simulink library "Phase2_Kinematics_Lib"  (R2026a)
settings: Solver=VariableStepAuto
settings Model: Creator=shueb  LastModifiedBy=shueb

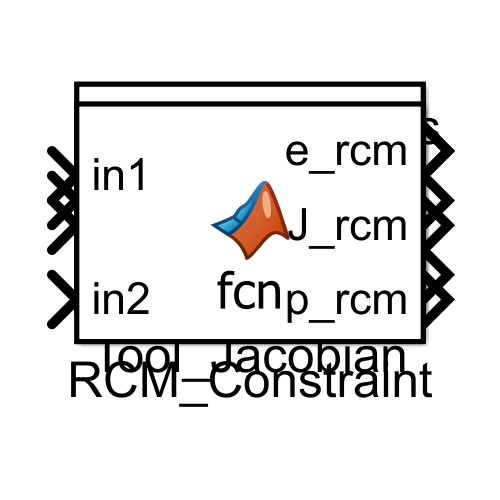
[thumbnail: Simulink's stored preview of the top-level diagram]
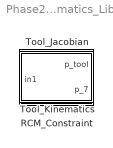
== system Phase2_Kinematics_Lib ==
  RCM_Constraint : MATLAB Function  TreatAsAtomicUnit=on
  Tool_Jacobian : MATLAB Function  TreatAsAtomicUnit=on
  Tool_Kinematics : MATLAB Function  TreatAsAtomicUnit=on

== matlab function Phase2_Kinematics_Lib/Tool_Jacobian ==
  data: in1 input; J_tool output
function J_tool = tool_jacobian(in1)
%#codegen

%    This function was generated by the Symbolic Math Toolbox version 26.1.
%    26-May-2026 08:31:23

% in1 = complex(in1);  % if required to enforce complex operations
q1 = in1(1,:);
q2 = in1(2,:);
q3 = in1(3,:);
q4 = in1(4,:);
q5 = in1(5,:);
q6 = in1(6,:);
t2 = cos(q1);
t3 = cos(q2);
t4 = cos(q3);
t5 = cos(q4);
t6 = cos(q5);
t7 = cos(q6);
t8 = sin(q1);
t9 = sin(q2);
t10 = sin(q3);
t11 = sin(q4);
t12 = sin(q5);
t13 = sin(q6);
t14 = t2.*t4;
t15 = t3.*t5;
t16 = t2.*t10;
t17 = t4.*t8;
t18 = t3.*t11;
t19 = t8.*t10;
t20 = t8.*t9.*t11;
t24 = t2.*t5.*t9;
t25 = t4.*t5.*t9;
t27 = t2.*t9.*t11;
t28 = t5.*t8.*t9;
t29 = t4.*t9.*t11;
t21 = t3.*t14;
t22 = t3.*t16;
t23 = t3.*t17;
t26 = t3.*t19;
t31 = -t25;
t37 = t15+t29;
t30 = -t21;
t32 = -t26;
t35 = t16+t23;
t36 = t17+t22;
t40 = t18+t31;
t38 = t14+t32;
t39 = t19+t30;
t41 = t5.*t35;
t42 = t11.*t35;
t43 = t12.*t36;
t44 = t5.*t39;
t45 = t11.*t39;
t46 = t12.*t38;
t47 = t20+t41;
t49 = t24+t45;
t50 = t6.*t47;
t52 = -t6.*(t27-t44);
t53 = t46+t50;
t54 = t43+t52;
mt1 = [t28.*(2.0./5.0)-t42.*(2.0./5.0)+t8.*t9.*(2.0./5.0)+t13.*t53.*(6.9e+1./2.5e+2)+t7.*(t28-t42).*(6.9e+1./2.5e+2),t24.*(-2.0./5.0)-t45.*(2.0./5.0)-t2.*t9.*(2.0./5.0)-t7.*t49.*(6.9e+1./2.5e+2)+t13.*t54.*(6.9e+1./2.5e+2),0.0,t13.*(t6.*(t2.*t18-t5.*t9.*t14)+t9.*t12.*t16).*(-6.9e+1./2.5e+2)-t7.*(t2.*t15+t9.*t11.*t14).*(6.9e+1./2.5e+2)-t2.*t3.*(2.0./5.0)-t2.*t15.*(2.0./5.0)-t9.*t11.*t14.*(2.0./5.0)];
mt2 = [t13.*(t6.*(t8.*t18-t5.*t9.*t17)+t9.*t12.*t19).*(-6.9e+1./2.5e+2)-t7.*(t8.*t15+t9.*t11.*t17).*(6.9e+1./2.5e+2)-t3.*t8.*(2.0./5.0)-t8.*t15.*(2.0./5.0)-t9.*t11.*t17.*(2.0./5.0),t9.*(-2.0./5.0)-t5.*t9.*(2.0./5.0)+t4.*t18.*(2.0./5.0)-t13.*(t6.*(t4.*t15+t9.*t11)-t3.*t10.*t12).*(6.9e+1./2.5e+2)-t7.*(t5.*t9-t4.*t18).*(6.9e+1./2.5e+2),t13.*(t12.*t39-t5.*t6.*t36).*(-6.9e+1./2.5e+2)-t11.*t36.*(2.0./5.0)-t7.*t11.*t36.*(6.9e+1./2.5e+2)];
mt3 = [t13.*(t12.*t35-t5.*t6.*t38).*(6.9e+1./2.5e+2)+t11.*t38.*(2.0./5.0)+t7.*t11.*t38.*(6.9e+1./2.5e+2),t13.*(t4.*t9.*t12+t5.*t6.*t9.*t10).*(6.9e+1./2.5e+2)-t9.*t10.*t11.*(2.0./5.0)-t7.*t9.*t10.*t11.*(6.9e+1./2.5e+2),t27.*(2.0./5.0)-t44.*(2.0./5.0)+t7.*(t27-t44).*(6.9e+1./2.5e+2)-t6.*t13.*t49.*(6.9e+1./2.5e+2),t20.*(2.0./5.0)+t41.*(2.0./5.0)+t7.*t47.*(6.9e+1./2.5e+2)-t6.*t13.*(t28-t42).*(6.9e+1./2.5e+2),t18.*(-2.0./5.0)+t25.*(2.0./5.0)-t7.*t40.*(6.9e+1./2.5e+2)+t6.*t13.*t37.*(6.9e+1./2.5e+2)];
mt4 = [t13.*(t6.*t36+t12.*(t27-t44)).*(6.9e+1./2.5e+2),t13.*(t6.*t38-t12.*t47).*(-6.9e+1./2.5e+2),t13.*(t12.*t40-t6.*t9.*t10).*(-6.9e+1./2.5e+2),t7.*t54.*(6.9e+1./2.5e+2)+t13.*t49.*(6.9e+1./2.5e+2),t7.*t53.*(-6.9e+1./2.5e+2)+t13.*(t28-t42).*(6.9e+1./2.5e+2),t7.*(t6.*t40+t9.*t10.*t12).*(6.9e+1./2.5e+2)-t13.*t37.*(6.9e+1./2.5e+2),0.0,0.0,0.0];
J_tool = reshape([mt1,mt2,mt3,mt4],3,7);
end

== matlab function Phase2_Kinematics_Lib/Tool_Kinematics ==
  data: in1 input; p_tool output; p_7 output
function [p_tool,p_7] = tool_kinematics(in1)
%#codegen

%    This function was generated by the Symbolic Math Toolbox version 26.1.
%    26-May-2026 08:31:21

% in1 = complex(in1);  % if required to enforce complex operations
q1 = in1(1,:);
q2 = in1(2,:);
q3 = in1(3,:);
q4 = in1(4,:);
q5 = in1(5,:);
q6 = in1(6,:);
t2 = cos(q1);
t3 = cos(q2);
t4 = cos(q3);
t5 = cos(q4);
t6 = cos(q5);
t7 = cos(q6);
t8 = sin(q1);
t9 = sin(q2);
t10 = sin(q3);
t11 = sin(q4);
t12 = sin(q5);
t13 = sin(q6);
t14 = t2.*t4;
t15 = t3.*t5;
t16 = t2.*t10;
t17 = t4.*t8;
t18 = t3.*t11;
t19 = t8.*t10;
t20 = t3.*(2.0./5.0);
t21 = t8.*t9.*t11;
t22 = t9.*t10.*t12;
t26 = t2.*t5.*t9;
t27 = t4.*t5.*t9;
t29 = t2.*t9.*t11;
t30 = t5.*t8.*t9;
t31 = t4.*t9.*t11;
t33 = t2.*t9.*(2.0./5.0);
t34 = t8.*t9.*(2.0./5.0);
t23 = t3.*t14;
t24 = t3.*t16;
t25 = t3.*t17;
t28 = t3.*t19;
t32 = t15.*(2.0./5.0);
t35 = -t33;
t36 = -t34;
t38 = -t27;
t42 = t26.*(2.0./5.0);
t43 = t30.*(2.0./5.0);
t44 = t31.*(2.0./5.0);
t49 = t15+t31;
t37 = -t23;
t39 = -t28;
t45 = -t42;
t46 = -t43;
t47 = t16+t25;
t48 = t17+t24;
t52 = t18+t38;
t50 = t14+t39;
t51 = t19+t37;
t53 = t5.*t47;
t54 = t11.*t47;
t55 = t12.*t48;
t57 = t6.*t52;
t56 = t5.*t51;
t58 = t11.*t51;
t59 = t12.*t50;
t60 = t54.*(2.0./5.0);
t63 = t21+t53;
t65 = t22+t57;
t61 = t58.*(2.0./5.0);
t66 = t26+t58;
t67 = t6.*t63;
t69 = -t6.*(t29-t56);
t62 = -t61;
t70 = t59+t67;
t71 = t55+t69;
p_tool = [t35+t45+t62-t7.*t66.*(6.9e+1./2.5e+2)+t13.*t71.*(6.9e+1./2.5e+2);t36+t46+t60-t13.*t70.*(6.9e+1./2.5e+2)-t7.*(t30-t54).*(6.9e+1./2.5e+2);t20+t32+t44+t7.*t49.*(6.9e+1./2.5e+2)+t13.*t65.*(6.9e+1./2.5e+2)];
if nargout > 1
    p_7 = [t35+t45+t62-t7.*t66.*(6.3e+1./5.0e+2)+t13.*t71.*(6.3e+1./5.0e+2);t36+t46+t60-t13.*t70.*(6.3e+1./5.0e+2)-t7.*(t30-t54).*(6.3e+1./5.0e+2);t20+t32+t44+t7.*t49.*(6.3e+1./5.0e+2)+t13.*t65.*(6.3e+1./5.0e+2)];
end
end

== matlab function Phase2_Kinematics_Lib/RCM_Constraint ==
  data: in1 input; e_rcm output; in2 input; J_rcm output; p_rcm output
function [e_rcm,J_rcm,p_rcm] = rcm_constraint(in1,in2)
%#codegen

%    This function was generated by the Symbolic Math Toolbox version 26.1.
%    26-May-2026 08:31:24

% in1 = complex(in1);  % if required to enforce complex operations
% in2 = complex(in2);  % if required to enforce complex operations
crx = in2(1,:);
cry = in2(2,:);
crz = in2(3,:);
q1 = in1(1,:);
q2 = in1(2,:);
q3 = in1(3,:);
q4 = in1(4,:);
q5 = in1(5,:);
q6 = in1(6,:);
t2 = cos(q1);
t3 = cos(q2);
t4 = cos(q3);
t5 = cos(q4);
t6 = cos(q5);
t7 = cos(q6);
t8 = sin(q1);
t9 = sin(q2);
t10 = sin(q3);
t11 = sin(q4);
t12 = sin(q5);
t13 = sin(q6);
t14 = -crz;
t15 = t2.*t4;
t16 = t3.*t5;
t17 = t2.*t10;
t18 = t4.*t8;
t19 = t3.*t11;
t20 = t5.*t9;
t21 = t8.*t10;
t22 = t9.*t11;
t23 = t3.*(2.0./5.0);
t24 = t9.*(2.0./5.0);
t26 = t9.*t10.*t12;
t42 = t3.*t10.*t12;
t43 = t4.*t9.*t12;
t44 = t6.*t9.*t10;
t52 = t2.*t9.*(-2.0./5.0);
t25 = t8.*t22;
t27 = t3.*t15;
t28 = t2.*t16;
t29 = t4.*t16;
t30 = t3.*t17;
t31 = t3.*t18;
t32 = t2.*t19;
t33 = t2.*t20;
t34 = t8.*t16;
t35 = t4.*t19;
t36 = t4.*t20;
t37 = t3.*t21;
t38 = t2.*t22;
t39 = t8.*t19;
t40 = t8.*t20;
t41 = t4.*t22;
t45 = t2.*t23;
t46 = t16.*(2.0./5.0);
t47 = t2.*t24;
t48 = t8.*t23;
t49 = t19.*(2.0./5.0);
t50 = t20.*(2.0./5.0);
t51 = t8.*t24;
t53 = t15.*t20;
t54 = t15.*t22;
t55 = t18.*t20;
t56 = t6.*t10.*t20;
t58 = t18.*t22;
t59 = t9.*t12.*t17;
t60 = t7.*t10.*t22;
t63 = t9.*t12.*t21;
t70 = t10.*t22.*(2.0./5.0);
t57 = -t27;
t61 = -t35;
t62 = -t36;
t64 = -t37;
t69 = t25.*(2.0./5.0);
t71 = t28.*(2.0./5.0);
t72 = t33.*(2.0./5.0);
t73 = t34.*(2.0./5.0);
t74 = t35.*(2.0./5.0);
t75 = t36.*(2.0./5.0);
t76 = t38.*(2.0./5.0);
t77 = t40.*(2.0./5.0);
t78 = t41.*(2.0./5.0);
t79 = -t53;
t80 = -t55;
t86 = t54.*(2.0./5.0);
t87 = t58.*(2.0./5.0);
t88 = t17+t31;
t89 = t18+t30;
t90 = t16+t41;
t91 = t22+t29;
t96 = t60.*(6.3e+1./5.0e+2);
t105 = t28+t54;
t106 = t34+t58;
t107 = t43+t56;
t82 = -t72;
t83 = -t74;
t84 = -t75;
t92 = t15+t64;
t93 = t21+t57;
t94 = t19+t62;
t95 = t20+t61;
t97 = t5.*t88;
t98 = t6.*t89;
t99 = t6.*t91;
t100 = t7.*t90;
t101 = t11.*t88;
t102 = t12.*t88;
t103 = t12.*t89;
t104 = t13.*t90;
t109 = t7.*t11.*t89;
t122 = t32+t79;
t123 = t39+t80;
t126 = t11.*t89.*(2.0./5.0);
t127 = t7.*t105;
t128 = t7.*t106;
t131 = t13.*t107;
t108 = t5.*t98;
t110 = t6.*t104;
t111 = t5.*t93;
t112 = t6.*t92;
t114 = t6.*t94;
t115 = t7.*t94;
t116 = t7.*t95;
t117 = t11.*t93;
t118 = t12.*t92;
t119 = t12.*t93;
t120 = t12.*t94;
t124 = t97.*(2.0./5.0);
t125 = t101.*(2.0./5.0);
t132 = t7.*t11.*t92;
t137 = t11.*t92.*(2.0./5.0);
t139 = t6.*t122;
t140 = t6.*t123;
t142 = t100.*(6.3e+1./5.0e+2);
t144 = t104.*(6.3e+1./5.0e+2);
t146 = t25+t97;
t147 = t109.*(6.3e+1./5.0e+2);
t154 = t127.*(6.3e+1./5.0e+2);
t155 = t128.*(6.3e+1./5.0e+2);
t156 = t131.*(6.3e+1./5.0e+2);
t170 = -t13.*(t42-t99);
t171 = -t13.*(t40-t101);
t183 = t7.*(t40-t101).*(-6.3e+1./5.0e+2);
t186 = t13.*(t42-t99).*(-6.3e+1./5.0e+2);
t187 = t13.*(t40-t101).*(-6.3e+1./5.0e+2);
t192 = t7.*(t40-t101).*(6.3e+1./5.0e+2);
t129 = t5.*t112;
t135 = -t125;
t136 = t111.*(2.0./5.0);
t138 = t117.*(2.0./5.0);
t145 = -t144;
t148 = t110.*(6.3e+1./5.0e+2);
t149 = t115.*(6.3e+1./5.0e+2);
t150 = t116.*(6.3e+1./5.0e+2);
t153 = t26+t114;
t157 = t132.*(6.3e+1./5.0e+2);
t158 = t33+t117;
t160 = t6.*t146;
t161 = t7.*t146;
t162 = t12.*t146;
t163 = -t156;
t174 = t6.*t171;
t175 = -t6.*(t38-t111);
t176 = -t7.*(t38-t111);
t178 = t59+t139;
t179 = t63+t140;
t194 = t6.*t187;
t202 = -t13.*(t108-t119);
t206 = t116+t170;
t210 = t13.*(t108-t119).*(-6.3e+1./5.0e+2);
t141 = -t129;
t143 = -t138;
t151 = -t148;
t166 = t7.*t158;
t168 = t13.*t158;
t169 = t7.*t153;
t172 = t13.*t153;
t181 = t161.*(6.3e+1./5.0e+2);
t189 = t13.*t178;
t190 = t13.*t179;
t203 = t118+t160;
t205 = t103+t175;
t218 = t70+t96+t163;
t227 = t161+t174;
t228 = t109+t202;
t238 = t24+t50+t83+t150+t186;
t241 = t126+t147+t210;
t173 = t6.*t168;
t182 = t166.*(6.3e+1./5.0e+2);
t184 = t168.*(6.3e+1./5.0e+2);
t185 = t169.*(6.3e+1./5.0e+2);
t188 = t172.*(6.3e+1./5.0e+2);
t196 = t102+t141;
t199 = t189.*(6.3e+1./5.0e+2);
t200 = t190.*(6.3e+1./5.0e+2);
t204 = t100+t172;
t211 = t7.*t203;
t212 = t13.*t203;
t214 = t7.*t205;
t215 = t13.*t205;
t221 = t127+t189;
t222 = t128+t190;
t231 = t49+t84+t149+t151;
t246 = t69+t124+t181+t194;
t191 = -t182;
t193 = t173.*(6.3e+1./5.0e+2);
t201 = t13.*t196;
t217 = -t215;
t219 = t211.*(6.3e+1./5.0e+2);
t220 = t212.*(6.3e+1./5.0e+2);
t223 = t214.*(6.3e+1./5.0e+2);
t224 = t215.*(6.3e+1./5.0e+2);
t226 = t145+t185;
t229 = t173+t176;
t232 = t171+t211;
t234 = t168+t214;
t237 = t13.*t204.*(t44-t120).*(6.3e+1./5.0e+2);
t239 = t14+t23+t46+t78+t142+t188;
t244 = t45+t71+t86+t154+t199;
t245 = t48+t73+t87+t155+t200;
t247 = t204.*t218;
t251 = t204.*(t144-t185);
t252 = t204.*t231;
t261 = t204.*t238;
t268 = t13.*(t212+t7.*(t40-t101)).*(t112-t162).*(6.3e+1./5.0e+2);
t209 = t201.*(6.3e+1./5.0e+2);
t225 = -t224;
t230 = t132+t201;
t236 = t166+t217;
t240 = t187+t219;
t242 = t184+t223;
t256 = t13.*t239.*(t44-t120);
t257 = -t239.*(t110-t115);
t259 = t51+t77+t135+t192+t220;
t263 = t204.*t239;
t265 = t206.*t239;
t267 = t239.*(t104-t169);
t243 = t137+t157+t209;
t260 = cry+t259;
t262 = t47+t72+t138+t182+t225;
t269 = t13.*t236.*(t98+t12.*(t38-t111)).*(-6.3e+1./5.0e+2);
t270 = -t240.*(t212+t7.*(t40-t101));
t271 = t236.*t241;
t272 = t236.*t242;
t275 = t236.*t244;
t295 = t236.*t259;
t264 = crx+t262;
t279 = t13.*t260.*(t112-t162);
t281 = t222.*t260;
t283 = t227.*t260;
t288 = t230.*t260;
t292 = t232.*t260;
t296 = -t262.*(t212+t7.*(t40-t101));
t297 = t236.*t260;
t298 = t260.*(t212+t7.*(t40-t101));
t280 = -t13.*t264.*(t98+t12.*(t38-t111));
t285 = t221.*t264;
t289 = t228.*t264;
t291 = t229.*t264;
t294 = -t292;
t299 = t234.*t264;
t301 = -t297;
t302 = t236.*t264;
t303 = t264.*(t212+t7.*(t40-t101));
t304 = t263+t298+t302;
t308 = t237+t256+t268+t269+t279+t280;
t309 = t295+t296+t301+t303;
t313 = t251+t267+t270+t272+t294+t299;
t305 = t204.*t304;
t306 = -t304.*(t212+t7.*(t40-t101));
t307 = t236.*t304;
e_rcm = [t264-t307;t260+t306;crz-t23-t46-t78-t142-t188+t305];
if nargout > 1
    mt1 = [t259+t306-t236.*t309,t52+t82+t143+t191+t224+t307-t309.*(t212+t7.*(t40-t101)),t204.*t309,-t71-t86-t154-t199-t2.*t3.*(2.0./5.0)+t221.*t304+t236.*(-t261-t265+t275+t281+t285+t245.*(t212+t7.*(t40-t101))),-t73-t87-t155-t200+(t212+t7.*(t40-t101)).*(-t261-t265+t275+t281+t285+t245.*(t212+t7.*(t40-t101)))-t3.*t8.*(2.0./5.0)+t222.*t304];
    mt2 = [-t24-t50+t74-t150+t206.*t304-t204.*(-t261-t265+t275+t281+t285+t245.*(t212+t7.*(t40-t101)))+t13.*(t42-t99).*(6.3e+1./5.0e+2),-t126-t147+t228.*t304-t236.*(t247-t271+t288-t289+t243.*(t212+t7.*(t40-t101))+t239.*(t60-t131))+t13.*(t108-t119).*(6.3e+1./5.0e+2),t243-(t212+t7.*(t40-t101)).*(t247-t271+t288-t289+t243.*(t212+t7.*(t40-t101))+t239.*(t60-t131))-t230.*t304];
    mt3 = [-t70-t96+t156+t204.*(t247-t271+t288-t289+t243.*(t212+t7.*(t40-t101))+t239.*(t60-t131))+t304.*(t60-t131),t76-t136-t193+t229.*t304-t236.*(t252+t257+t283-t291+t246.*(t212+t7.*(t40-t101))+t236.*(t76-t136-t193+t7.*(t38-t111).*(6.3e+1./5.0e+2)))+t7.*(t38-t111).*(6.3e+1./5.0e+2),t246-(t212+t7.*(t40-t101)).*(t252+t257+t283-t291+t246.*(t212+t7.*(t40-t101))+t236.*(t76-t136-t193+t7.*(t38-t111).*(6.3e+1./5.0e+2)))-t227.*t304];
    mt4 = [-t49+t75+t148-t149+t204.*(t252+t257+t283-t291+t246.*(t212+t7.*(t40-t101))+t236.*(t76-t136-t193+t7.*(t38-t111).*(6.3e+1./5.0e+2)))-t304.*(t110-t115),t13.*(t98+t12.*(t38-t111)).*(6.3e+1./5.0e+2)+t236.*t308-t13.*t304.*(t98+t12.*(t38-t111)),t308.*(t212+t7.*(t40-t101))-t13.*(t112-t162).*(6.3e+1./5.0e+2)+t13.*t304.*(t112-t162),-t204.*t308+t13.*(t44-t120).*(6.3e+1./5.0e+2)-t13.*t304.*(t44-t120),t242-t234.*t304-t236.*t313];
    mt5 = [-t219-t313.*(t212+t7.*(t40-t101))+t232.*t304+t13.*(t40-t101).*(6.3e+1./5.0e+2),t226+t204.*t313+t304.*(t104-t169),0.0,0.0,0.0];
    J_rcm = reshape([mt1,mt2,mt3,mt4,mt5],3,7);
end
if nargout > 2
    p_rcm = [t52+t82+t143+t191+t224+t307;-t77+t125+t183-t220+t304.*(t212+t7.*(t40-t101))-t8.*t9.*(2.0./5.0);t23+t46+t78+t142+t188-t305];
end
end
